simulink model "ballbeam_sim2"  (R2015a)
settings: Solver=ode45  StartTime=0.0  StopTime=200  RelTol=1e-3
InitFcn:
  | param
undefined symbols (not defined in the file or in its folder): drawBallBeam, P
settings Model: Creator=beard  LastModifiedBy=wynn4
settings DataIOCC: SignalLoggingSaveFormat=ModelDataLogs
settings OptimizationCC: ExpressionDepthLimit=2147483647  InitFltsAndDblsToZero=on
settings DebuggingCC: UnderspecifiedInitializationDetection=Classic  MergeDetectMultiDrivingBlocksExec=none  SolverPrmCheckMsg=warning  FcnCallInpInsideContextMsg=UseLocalSettings  StateNameClashWarn=warning
settings GRTTargetCC: CombineOutputUpdateFcns=off  GRTInterface=on

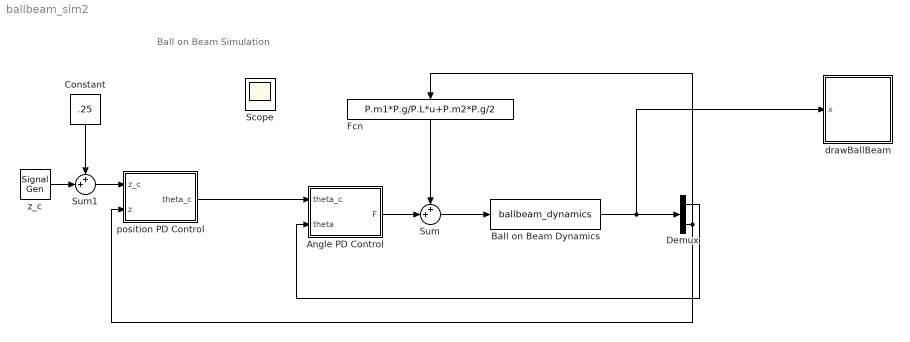
== system ballbeam_sim2 ==
  note: Ball on Beam Simulation
  "Angle PD Control " : Subsystem
  Ball on Beam Dynamics : S-Function  FunctionName=ballbeam_dynamics  Parameters=AP
  Constant : Constant  Value=.25
  Demux : Demux  Outputs=2
  Fcn : Fcn  Expr=P.m1*P.g/P.L*u+P.m2*P.g/2
  Scope : Scope
      settings: YMin=-0.003  YMax=0.001  SaveName=ScopeData2
  Sum : Sum  Inputs=++|
  Sum1 : Sum  Inputs=++|
  drawBallBeam : Subsystem
      mask Display: image(imread('tv.jpg'))
  position PD Control : Subsystem
  z_c : SignalGenerator  WaveForm=square  Amplitude=.15  Frequency=.01
  wires:
  Ball on Beam Dynamics/1 -> drawBallBeam/1(x), Demux/1
  position PD Control/1(theta_c) -> "Angle PD Control "/1(theta_c)
  Demux/2 -> Fcn/1, position PD Control/2(z)
  Demux/1 -> "Angle PD Control "/2(theta)
  Sum/1 -> Ball on Beam Dynamics/1
  Fcn/1 -> Sum/1
  "Angle PD Control "/1(F) -> Sum/2
  z_c/1 -> Sum1/2
  Sum1/1 -> position PD Control/1(z_c)
  Constant/1 -> Sum1/1

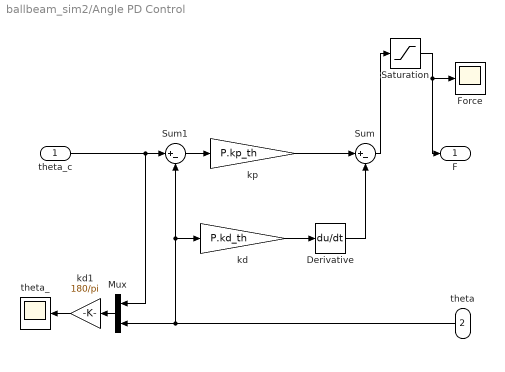
== system ballbeam_sim2/Angle PD Control  ==
  theta_c : Inport
  theta : Inport  Port=2
  Derivative : Derivative
  Force : Scope
      settings: YMin=-8e-05  YMax=4e-05
  Mux : Mux  Inputs=2
  Saturation : Saturate  UpperLimit=15  LowerLimit=-15
  Sum : Sum  Inputs=|+-
  Sum1 : Sum  Inputs=|+-
  kd : Gain  Gain=P.kd_th
  kd1 : Gain  Gain=180/pi
  kp : Gain  Gain=P.kp_th
  theta_ : Scope
      settings: TimeRange=200  YMin=-0.1  YMax=0.1
  F : Outport
  wires:
  Derivative/1 -> Sum/2
  kd/1 -> Derivative/1
  Mux/1 -> kd1/1
  kp/1 -> Sum/1
  kd1/1 -> theta_/1
  Sum1/1 -> kp/1
  theta/1 -> Mux/2, Sum1/2, kd/1
  theta_c/1 -> Mux/1, Sum1/1
  Sum/1 -> Saturation/1
  Saturation/1 -> Force/1, F/1

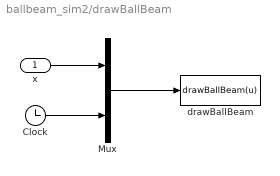
== system ballbeam_sim2/drawBallBeam ==
  x : Inport
  Clock : Clock
  Mux : Mux  Inputs=2
  drawBallBeam : MATLABFcn  MATLABFcn=drawBallBeam(u)  OutputDimensions=0  SampleTime=0.1
  wires:
  Mux/1 -> drawBallBeam/1
  x/1 -> Mux/1
  Clock/1 -> Mux/2

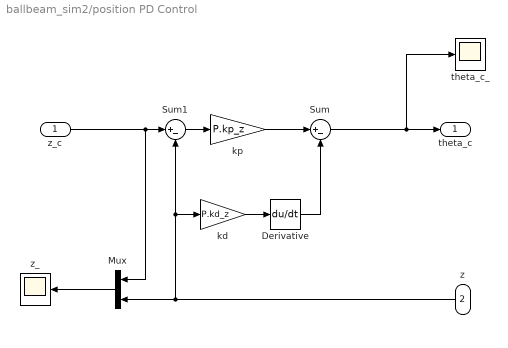
== system ballbeam_sim2/position PD Control ==
  z_c : Inport
  z : Inport  Port=2
  Derivative : Derivative
  Mux : Mux  Inputs=2
  Sum : Sum  Inputs=|+-
  Sum1 : Sum  Inputs=|+-
  kd : Gain  Gain=P.kd_z
  kp : Gain  Gain=P.kp_z
  theta_c_ : Scope
      settings: YMin=0.15  YMax=1
  z_ : Scope
      settings: TimeRange=200  YMin=-0.05  YMax=0.55
  theta_c : Outport
  wires:
  Derivative/1 -> Sum/2
  kd/1 -> Derivative/1
  kp/1 -> Sum/1
  Mux/1 -> z_/1
  Sum1/1 -> kp/1
  z/1 -> Mux/2, Sum1/2, kd/1
  Sum/1 -> theta_c/1, theta_c_/1
  z_c/1 -> Mux/1, Sum1/1
